simulink model "PVRobusMPC_final"  (R2018a)
settings: Solver=ode2  StartTime=0.0  StopTime=43200  FixedStep=1  RelTol=1e-3  EnableMultiTasking=on
InitFcn:
  | load PV_model_data
StopFcn:
  | save results Lambda_UV01 T_PV_Reference Tm_f01 Pout01 Tamb Time
  | clear all
  | load results
  | figure
  | subplot(3,1,1)
  | plot(Time./3600,T_PV_Reference,Time./3600,Tm_f01)
  | legend('PV Temperature Reference','PV Temperature')
  | title('MPC Tracking')
  | ylim([350 380])
  | subplot(3,1,2)
  | plot(Time./3600,Lambda_UV01)
  | ylim([250 450])
  | legend('\lambda_U_V')
  | subplot(3,1,3)
  | plot(Time./3600,Pout01)
  | legend('PV Power')
  | xlabel('Time [hours]')
  | ylabel('Watt')
values from neighbouring files (symbols this model uses):
  Global_tilt_Irr_2_2_12_13_5 = [0.000279 0.000786 0.00115 0.00401 0.0047 0.0102 0.011 0.0195 0.0266 0.0299 0.0338 0.0682 ... (2802 elements, 1401x2)]    [PV_model_data.mat]
  Total_light_absorption_in_polystyren = [0.0148235487596 0.0159326919994 0.0170383922491 0.0181406655151 0.0192395277052 0.0203349946285 0.0214270819969 0.0225158054254 0.0236011804327 0.0246832224425 0.0257619467839 0.0264640052027 ... (1151 elements, 1151x1)]    [PV_model_data.mat]
  Total_light_absorption_in_PV_cell_acrylic = [0.0222539070262 0.0239185757929 0.0255780524095 0.0272323791236 0.0288816001883 0.030525761736 0.0321649116541 0.0337990994657 0.0354283762117 0.0370527943369 0.0386724075795 0.0397267002838 ... (1151 elements, 1151x1)]    [PV_model_data.mat]
libraries: mpclib x256
(part 1 of 72)
settings Model: Creator=hg212  LastModifiedBy=Mehdi
settings DataIOCC: LimitDataPoints=on  SaveFormat=Array  SignalLoggingSaveFormat=ModelDataLogs
settings OptimizationCC: LifeSpan=inf
settings DebuggingCC: FcnCallInpInsideContextMsg=warning  SFUnexpectedBacktrackingDiag=warning  SFNoUnconditionalDefaultTransitionDiag=warning  SFExecutionAtInitializationDiag=none
settings HardwareCC: ProdBitPerPointer=32  ProdBitPerSizeT=32  ProdBitPerPtrDiffT=32  ProdLargestAtomicFloat=None  ProdIntDivRoundTo=Undefined  ProdEndianess=Unspecified  ProdWordSize=32  ProdHWDeviceType=32-bit Generic
settings ModelReferenceCC: PropagateSignalLabelsOutOfModel=off
settings CodeAppCC: StateflowObjectComments=on
settings GRTTargetCC: TargetLangStandard=C89/C90 (ANSI)  GeneratePreprocessorConditionals=Disable all  CombineOutputUpdateFcns=off  GRTInterface=on
settings ConfigComp: CovMetricSettings=dw  CovHtmlReporting=on  CovSaveCumulativeToWorkspaceVar=on  CovSaveSingleToWorkspaceVar=on  CovExternalEMLEnable=off

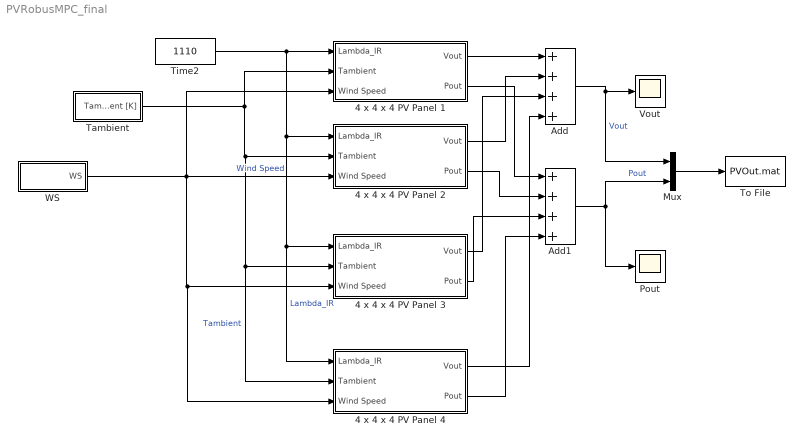
== system PVRobusMPC_final ==
  4 x 4 x 4 PV Panel 1 : Subsystem
  4 x 4 x 4 PV Panel 2 : Subsystem
  4 x 4 x 4 PV Panel 3 : Subsystem
  4 x 4 x 4 PV Panel 4 : Subsystem
  Add : Sum  Inputs=++++
  Add1 : Sum  Inputs=++++
  Mux : Mux  Inputs=2
  Pout : Scope
  Tambient : Subsystem
  Time2 : Constant  Value=1110
  To File : ToFile  Filename=PVOut.mat  SaveFormat=Timeseries
  Vout : Scope
  WS : Subsystem
  wires:
  Time2/1 -> 4 x 4 x 4 PV Panel 4/1(Lambda_IR), 4 x 4 x 4 PV Panel 3/1(Lambda_IR), 4 x 4 x 4 PV Panel 2/1(Lambda_IR), 4 x 4 x 4 PV Panel 1/1(Lambda_IR)  "Lambda_IR"
  Tambient/1(Tambient [K]) -> 4 x 4 x 4 PV Panel 1/2(Tambient), 4 x 4 x 4 PV Panel 4/2(Tambient), 4 x 4 x 4 PV Panel 3/2(Tambient), 4 x 4 x 4 PV Panel 2/2(Tambient)  "Tambient"
  WS/1(WS) -> 4 x 4 x 4 PV Panel 4/3(Wind Speed), 4 x 4 x 4 PV Panel 3/3(Wind Speed), 4 x 4 x 4 PV Panel 2/3(Wind Speed), 4 x 4 x 4 PV Panel 1/3(Wind Speed)  "Wind Speed"
  4 x 4 x 4 PV Panel 1/1(Vout) -> Add/1
  4 x 4 x 4 PV Panel 2/1(Vout) -> Add/2
  4 x 4 x 4 PV Panel 1/2(Pout) -> Add1/1
  4 x 4 x 4 PV Panel 2/2(Pout) -> Add1/2
  Add/1 -> Mux/1, Vout/1  "Vout"
  Add1/1 -> Pout/1, Mux/2  "Pout"
  Mux/1 -> To File/1
  4 x 4 x 4 PV Panel 3/1(Vout) -> Add/3
  4 x 4 x 4 PV Panel 4/1(Vout) -> Add/4
  4 x 4 x 4 PV Panel 3/2(Pout) -> Add1/3
  4 x 4 x 4 PV Panel 4/2(Pout) -> Add1/4

== system PVRobusMPC_final/4 x 4 x 4 PV Panel 1 ==
  Lambda_IR : Inport
  Tambient : Inport  Port=2
  Wind Speed : Inport  Port=3
  4 x 4 PV Panel 1 : Subsystem
  4 x 4 PV Panel 2 : Subsystem
  4 x 4 PV Panel 3 : Subsystem
  4 x 4 PV Panel 4 : Subsystem
  Add : Sum  Inputs=++++
  Add1 : Sum  Inputs=++++
  Vout : Outport
  Pout : Outport  Port=2
  wires:
  4 x 4 PV Panel 2/1(Vout) -> Add/2
  4 x 4 PV Panel 2/2(Pout) -> Add1/2
  4 x 4 PV Panel 4/1(Vout) -> Add/4
  Tambient/1 -> 4 x 4 PV Panel 2/2(Tambient), 4 x 4 PV Panel 4/2(Tambient), 4 x 4 PV Panel 3/2(Tambient), 4 x 4 PV Panel 1/2(Tambient)
  Add1/1 -> Pout/1
  4 x 4 PV Panel 3/1(Vout) -> Add/3
  Lambda_IR/1 -> 4 x 4 PV Panel 4/1(Lambda_IR), 4 x 4 PV Panel 3/1(Lambda_IR), 4 x 4 PV Panel 2/1(Lambda_IR), 4 x 4 PV Panel 1/1(Lambda_IR)
  4 x 4 PV Panel 1/1(Vout) -> Add/1
  4 x 4 PV Panel 4/2(Pout) -> Add1/4
  Wind Speed/1 -> 4 x 4 PV Panel 2/3(Wind Speed), 4 x 4 PV Panel 4/3(Wind Speed), 4 x 4 PV Panel 3/3(Wind Speed), 4 x 4 PV Panel 1/3(Wind Speed)
  4 x 4 PV Panel 3/2(Pout) -> Add1/3
  4 x 4 PV Panel 1/2(Pout) -> Add1/1
  Add/1 -> Vout/1

== system PVRobusMPC_final/4 x 4 x 4 PV Panel 2 ==
  Lambda_IR : Inport
  Tambient : Inport  Port=2
  Wind Speed : Inport  Port=3
  4 x 4 PV Panel 5 : Subsystem
  4 x 4 PV Panel 6 : Subsystem
  4 x 4 PV Panel 7 : Subsystem
  4 x 4 PV Panel 8 : Subsystem
  Add2 : Sum  Inputs=++++
  Add3 : Sum  Inputs=++++
  Vout : Outport
  Pout : Outport  Port=2
  wires:
  Wind Speed/1 -> 4 x 4 PV Panel 8/3(Wind Speed), 4 x 4 PV Panel 7/3(Wind Speed), 4 x 4 PV Panel 6/3(Wind Speed), 4 x 4 PV Panel 5/3(Wind Speed)
  Add3/1 -> Pout/1
  Add2/1 -> Vout/1
  4 x 4 PV Panel 6/1(Vout) -> Add2/2
  Lambda_IR/1 -> 4 x 4 PV Panel 8/1(Lambda_IR), 4 x 4 PV Panel 7/1(Lambda_IR), 4 x 4 PV Panel 6/1(Lambda_IR), 4 x 4 PV Panel 5/1(Lambda_IR)
  Tambient/1 -> 4 x 4 PV Panel 8/2(Tambient), 4 x 4 PV Panel 7/2(Tambient), 4 x 4 PV Panel 6/2(Tambient), 4 x 4 PV Panel 5/2(Tambient)
  4 x 4 PV Panel 8/1(Vout) -> Add2/4
  4 x 4 PV Panel 6/2(Pout) -> Add3/2
  4 x 4 PV Panel 5/1(Vout) -> Add2/1
  4 x 4 PV Panel 7/1(Vout) -> Add2/3
  4 x 4 PV Panel 5/2(Pout) -> Add3/1
  4 x 4 PV Panel 7/2(Pout) -> Add3/3
  4 x 4 PV Panel 8/2(Pout) -> Add3/4

== system PVRobusMPC_final/4 x 4 x 4 PV Panel 3 ==
  Lambda_IR : Inport
  Tambient : Inport  Port=2
  Wind Speed : Inport  Port=3
  4 x 4 PV Panel 5 : Subsystem
  4 x 4 PV Panel 6 : Subsystem
  4 x 4 PV Panel 7 : Subsystem
  4 x 4 PV Panel 8 : Subsystem
  Add2 : Sum  Inputs=++++
  Add3 : Sum  Inputs=++++
  Vout : Outport
  Pout : Outport  Port=2
  wires:
  4 x 4 PV Panel 8/2(Pout) -> Add3/4
  4 x 4 PV Panel 7/2(Pout) -> Add3/3
  4 x 4 PV Panel 5/2(Pout) -> Add3/1
  4 x 4 PV Panel 7/1(Vout) -> Add2/3
  4 x 4 PV Panel 5/1(Vout) -> Add2/1
  4 x 4 PV Panel 6/2(Pout) -> Add3/2
  4 x 4 PV Panel 8/1(Vout) -> Add2/4
  Tambient/1 -> 4 x 4 PV Panel 5/2(Tambient), 4 x 4 PV Panel 6/2(Tambient), 4 x 4 PV Panel 7/2(Tambient), 4 x 4 PV Panel 8/2(Tambient)
  Lambda_IR/1 -> 4 x 4 PV Panel 5/1(Lambda_IR), 4 x 4 PV Panel 6/1(Lambda_IR), 4 x 4 PV Panel 7/1(Lambda_IR), 4 x 4 PV Panel 8/1(Lambda_IR)
  4 x 4 PV Panel 6/1(Vout) -> Add2/2
  Add2/1 -> Vout/1
  Add3/1 -> Pout/1
  Wind Speed/1 -> 4 x 4 PV Panel 5/3(Wind Speed), 4 x 4 PV Panel 6/3(Wind Speed), 4 x 4 PV Panel 7/3(Wind Speed), 4 x 4 PV Panel 8/3(Wind Speed)

== system PVRobusMPC_final/4 x 4 x 4 PV Panel 4 ==
  Lambda_IR : Inport
  Tambient : Inport  Port=2
  Wind Speed : Inport  Port=3
  4 x 4 PV Panel 5 : Subsystem
  4 x 4 PV Panel 6 : Subsystem
  4 x 4 PV Panel 7 : Subsystem
  4 x 4 PV Panel 8 : Subsystem
  Add2 : Sum  Inputs=++++
  Add3 : Sum  Inputs=++++
  Vout : Outport
  Pout : Outport  Port=2
  wires:
  Wind Speed/1 -> 4 x 4 PV Panel 8/3(Wind Speed), 4 x 4 PV Panel 7/3(Wind Speed), 4 x 4 PV Panel 6/3(Wind Speed), 4 x 4 PV Panel 5/3(Wind Speed)
  Add3/1 -> Pout/1
  Add2/1 -> Vout/1
  4 x 4 PV Panel 6/1(Vout) -> Add2/2
  Lambda_IR/1 -> 4 x 4 PV Panel 8/1(Lambda_IR), 4 x 4 PV Panel 7/1(Lambda_IR), 4 x 4 PV Panel 6/1(Lambda_IR), 4 x 4 PV Panel 5/1(Lambda_IR)
  Tambient/1 -> 4 x 4 PV Panel 8/2(Tambient), 4 x 4 PV Panel 7/2(Tambient), 4 x 4 PV Panel 6/2(Tambient), 4 x 4 PV Panel 5/2(Tambient)
  4 x 4 PV Panel 8/1(Vout) -> Add2/4
  4 x 4 PV Panel 6/2(Pout) -> Add3/2
  4 x 4 PV Panel 5/1(Vout) -> Add2/1
  4 x 4 PV Panel 7/1(Vout) -> Add2/3
  4 x 4 PV Panel 5/2(Pout) -> Add3/1
  4 x 4 PV Panel 7/2(Pout) -> Add3/3
  4 x 4 PV Panel 8/2(Pout) -> Add3/4

== system PVRobusMPC_final/Tambient ==
  1-D Lookup Table2 : Lookup_n-D  NumberOfTableDimensions=1  BreakpointsForDimension1=0:600:144*600  Table="[18.16\t18.09\t17.96\t17.97\t18.07\t18.01\t17.98\t17.87\t17.72\t17.76\t17.8\t17.7\t17.54\t17.55\t17.41\t17.38\t17.34\t17.47\t17.23\t17.27\t17.23\t17.29\t17.27\t17.32\t17.27\t17.31\t17.25\t17.48\t17.42\t17.19\t17.16\t17.27\t17.02\t17.11\t17.16\t17.33\t17.27\t17.02\t17\t16.95\t16.96\t16.94\t16.8\t16.73\t16.57\t16.42\t16.64\t16.68\t16.7\t16.94\t17.23\t17.51\t17.41\t17.47\t17.5\t17.69\t17.69\t18.18\t17.97\t17.71\t17.72\t17.83\t18.18\t18.64\t18.99\t18.7\t18.92\t18.9\t19.85\t20.72\t20.99\t20.74\t20.32\t20.88\t21.21\t20.34\t21.6\t20.68\t21.32\t22\t20.4\t21.32\t20.42\t20.54\t22.31\t21.62\t21.9\t20.73\t21.21\t22.06\t22.15\t21.67\t22.11\t21.42\t22.21\t22.47\t23.13\t22.24\t22.02\t21.92\t21.14\t21.67\t21.89\t22.18\t22.28\t21.16\t22.06\t20.81\t20.78\t21.13\t21.15\t20.81\t20.83\t21.02\t20.89\t20.71\t20.73\t20.45\t20.42\t20.09\t20.26\t19.9\t19.45\t19.31\t19.32\t19.1\t18.94\t18.94\t18.8\t18.72\t18.59\t18.5\t18.44\t18.49\t18.46\t18.45\t18.56\t18.32\t18.08\t17.93\t17.79\t17.56\t17.54\t17.23\t17.07]+30+273"  InternalRulePriority=Speed  RndMeth=Simplest  InputSameDT=on
  Clock : Clock
  To Workspace3 : ToWorkspace  VariableName=Tamb  SampleTime=1
  To Workspace7 : ToWorkspace  VariableName=Time  SampleTime=1
  Tambient [K] : Outport
  wires:
  1-D Lookup Table2/1 -> Tambient [K]/1, To Workspace3/1
  Clock/1 -> To Workspace7/1, 1-D Lookup Table2/1

== system PVRobusMPC_final/WS ==
  1-D Lookup Table3 : Lookup_n-D  NumberOfTableDimensions=1  BreakpointsForDimension1=0:600:144*600  Table="[8\t7\t8\t7\t7\t8\t7\t7\t5\t6\t7\t7\t7\t7\t6\t7\t6\t7\t6\t5\t5\t6\t6\t5\t6\t6\t7\t7\t7\t6\t6\t6\t6\t6\t6\t7\t7\t7\t6\t7\t5\t6\t7\t6\t6\t5\t7\t7\t5\t5\t6\t6\t7\t7\t7\t7\t7\t7\t6\t6\t7\t7\t6\t7\t7\t7\t7\t7\t7\t8\t8\t8\t8\t7\t8\t7\t8\t9\t8\t7\t8\t7\t8\t6\t9\t9\t9\t10\t7\t8\t8\t8\t9\t8\t9\t9\t8\t9\t8\t9\t9\t7\t8\t8\t8\t9\t8\t8\t8\t8\t7\t8\t7\t8\t7\t7\t7\t8\t8\t8\t7\t7\t8\t7\t7\t6\t6\t7\t6\t5\t6\t6\t6\t5\t5\t5\t6\t6\t5\t5\t5\t4\t5\t4\t4].*0.277/5"  InternalRulePriority=Speed  RndMeth=Simplest  InputSameDT=on
  Clock1 : Clock
  To Workspace4 : ToWorkspace  VariableName=WS  SampleTime=1
  WS : Outport
  wires:
  Clock1/1 -> 1-D Lookup Table3/1
  1-D Lookup Table3/1 -> WS/1, To Workspace4/1

== system PVRobusMPC_final/4 x 4 x 4 PV Panel 1/4 x 4 PV Panel 1 ==
  Lambda_IR : Inport
  Tambient : Inport  Port=2
  Wind Speed : Inport  Port=3
  4 PV Panel 1 : Subsystem
  4 PV Panel 2 : Subsystem
  4 PV Panel 3 : Subsystem
  4 PV Panel 4 : Subsystem
  Add : Sum  Inputs=++++
  Add2 : Sum  Inputs=++++
  Vout : Outport
  Pout : Outport  Port=2
  wires:
  Wind Speed/1 -> 4 PV Panel 1/3(Wind Speed), 4 PV Panel 2/3(Wind Speed), 4 PV Panel 4/3(Wind Speed), 4 PV Panel 3/3(Wind Speed)
  4 PV Panel 3/2(Pout) -> Add2/3
  4 PV Panel 4/2(Pout) -> Add2/4
  4 PV Panel 3/1(Vout) -> Add/3
  4 PV Panel 2/2(Pout) -> Add2/2
  4 PV Panel 1/1(Vout) -> Add/1
  4 PV Panel 1/2(Pout) -> Add2/1
  Lambda_IR/1 -> 4 PV Panel 4/1(lambda_IR), 4 PV Panel 3/1(lambda_IR), 4 PV Panel 2/1(lambda_IR), 4 PV Panel 1/1(lambda_IR)
  4 PV Panel 4/1(Vout) -> Add/4
  Tambient/1 -> 4 PV Panel 1/2(Tambient1), 4 PV Panel 4/2(Tambient), 4 PV Panel 3/2(Tambient), 4 PV Panel 2/2(Tambient)
  4 PV Panel 2/1(Vout) -> Add/2
  Add2/1 -> Pout/1
  Add/1 -> Vout/1

== system PVRobusMPC_final/4 x 4 x 4 PV Panel 1/4 x 4 PV Panel 2 ==
  Lambda_IR : Inport
  Tambient : Inport  Port=2
  Wind Speed : Inport  Port=3
  4 PV Panel 1 : Subsystem
  4 PV Panel 2 : Subsystem
  4 PV Panel 3 : Subsystem
  4 PV Panel 4 : Subsystem
  Add : Sum  Inputs=++++
  Add2 : Sum  Inputs=++++
  Vout : Outport
  Pout : Outport  Port=2
  wires:
  Add/1 -> Vout/1
  Add2/1 -> Pout/1
  4 PV Panel 2/1(Vout) -> Add/2
  Tambient/1 -> 4 PV Panel 2/2(Tambient), 4 PV Panel 3/2(Tambient), 4 PV Panel 4/2(Tambient), 4 PV Panel 1/2(Tambient1)
  4 PV Panel 4/1(Vout) -> Add/4
  Lambda_IR/1 -> 4 PV Panel 1/1(lambda_IR), 4 PV Panel 2/1(lambda_IR), 4 PV Panel 3/1(lambda_IR), 4 PV Panel 4/1(lambda_IR)
  4 PV Panel 1/2(Pout) -> Add2/1
  4 PV Panel 1/1(Vout) -> Add/1
  4 PV Panel 2/2(Pout) -> Add2/2
  4 PV Panel 3/1(Vout) -> Add/3
  4 PV Panel 4/2(Pout) -> Add2/4
  4 PV Panel 3/2(Pout) -> Add2/3
  Wind Speed/1 -> 4 PV Panel 3/3(Wind Speed), 4 PV Panel 4/3(Wind Speed), 4 PV Panel 2/3(Wind Speed), 4 PV Panel 1/3(Wind Speed)

== system PVRobusMPC_final/4 x 4 x 4 PV Panel 1/4 x 4 PV Panel 3 ==
  Lambda_IR : Inport
  Tambient : Inport  Port=2
  Wind Speed : Inport  Port=3
  4 PV Panel 1 : Subsystem
  4 PV Panel 2 : Subsystem
  4 PV Panel 3 : Subsystem
  4 PV Panel 4 : Subsystem
  Add : Sum  Inputs=++++
  Add2 : Sum  Inputs=++++
  Vout : Outport
  Pout : Outport  Port=2
  wires:
  Add/1 -> Vout/1
  Add2/1 -> Pout/1
  4 PV Panel 2/1(Vout) -> Add/2
  Tambient/1 -> 4 PV Panel 2/2(Tambient), 4 PV Panel 3/2(Tambient), 4 PV Panel 4/2(Tambient), 4 PV Panel 1/2(Tambient1)
  4 PV Panel 4/1(Vout) -> Add/4
  Lambda_IR/1 -> 4 PV Panel 1/1(lambda_IR), 4 PV Panel 2/1(lambda_IR), 4 PV Panel 3/1(lambda_IR), 4 PV Panel 4/1(lambda_IR)
  4 PV Panel 1/2(Pout) -> Add2/1
  4 PV Panel 1/1(Vout) -> Add/1
  4 PV Panel 2/2(Pout) -> Add2/2
  4 PV Panel 3/1(Vout) -> Add/3
  4 PV Panel 4/2(Pout) -> Add2/4
  4 PV Panel 3/2(Pout) -> Add2/3
  Wind Speed/1 -> 4 PV Panel 3/3(Wind Speed), 4 PV Panel 4/3(Wind Speed), 4 PV Panel 2/3(Wind Speed), 4 PV Panel 1/3(Wind Speed)

== system PVRobusMPC_final/4 x 4 x 4 PV Panel 1/4 x 4 PV Panel 4 ==
  Lambda_IR : Inport
  Tambient : Inport  Port=2
  Wind Speed : Inport  Port=3
  4 PV Panel 1 : Subsystem
  4 PV Panel 2 : Subsystem
  4 PV Panel 3 : Subsystem
  4 PV Panel 4 : Subsystem
  Add : Sum  Inputs=++++
  Add2 : Sum  Inputs=++++
  Vout : Outport
  Pout : Outport  Port=2
  wires:
  Add/1 -> Vout/1
  Add2/1 -> Pout/1
  4 PV Panel 2/1(Vout) -> Add/2
  Tambient/1 -> 4 PV Panel 2/2(Tambient), 4 PV Panel 3/2(Tambient), 4 PV Panel 4/2(Tambient), 4 PV Panel 1/2(Tambient1)
  4 PV Panel 4/1(Vout) -> Add/4
  Lambda_IR/1 -> 4 PV Panel 1/1(lambda_IR), 4 PV Panel 2/1(lambda_IR), 4 PV Panel 3/1(lambda_IR), 4 PV Panel 4/1(lambda_IR)
  4 PV Panel 1/2(Pout) -> Add2/1
  4 PV Panel 1/1(Vout) -> Add/1
  4 PV Panel 2/2(Pout) -> Add2/2
  4 PV Panel 3/1(Vout) -> Add/3
  4 PV Panel 4/2(Pout) -> Add2/4
  4 PV Panel 3/2(Pout) -> Add2/3
  Wind Speed/1 -> 4 PV Panel 3/3(Wind Speed), 4 PV Panel 4/3(Wind Speed), 4 PV Panel 2/3(Wind Speed), 4 PV Panel 1/3(Wind Speed)

== system PVRobusMPC_final/4 x 4 x 4 PV Panel 2/4 x 4 PV Panel 5 ==
  Lambda_IR : Inport
  Tambient : Inport  Port=2
  Wind Speed : Inport  Port=3
  4 PV Panel 1 : Subsystem
  4 PV Panel 2 : Subsystem
  4 PV Panel 3 : Subsystem
  4 PV Panel 4 : Subsystem
  Add : Sum  Inputs=++++
  Add2 : Sum  Inputs=++++
  Vout : Outport
  Pout : Outport  Port=2
  wires:
  Wind Speed/1 -> 4 PV Panel 1/3(Wind Speed), 4 PV Panel 2/3(Wind Speed), 4 PV Panel 4/3(Wind Speed), 4 PV Panel 3/3(Wind Speed)
  4 PV Panel 3/2(Pout) -> Add2/3
  4 PV Panel 4/2(Pout) -> Add2/4
  4 PV Panel 3/1(Vout) -> Add/3
  4 PV Panel 2/2(Pout) -> Add2/2
  4 PV Panel 1/1(Vout) -> Add/1
  4 PV Panel 1/2(Pout) -> Add2/1
  Lambda_IR/1 -> 4 PV Panel 4/1(lambda_IR), 4 PV Panel 3/1(lambda_IR), 4 PV Panel 2/1(lambda_IR), 4 PV Panel 1/1(lambda_IR)
  4 PV Panel 4/1(Vout) -> Add/4
  Tambient/1 -> 4 PV Panel 1/2(Tambient1), 4 PV Panel 4/2(Tambient), 4 PV Panel 3/2(Tambient), 4 PV Panel 2/2(Tambient)
  4 PV Panel 2/1(Vout) -> Add/2
  Add2/1 -> Pout/1
  Add/1 -> Vout/1

== system PVRobusMPC_final/4 x 4 x 4 PV Panel 2/4 x 4 PV Panel 6 ==
  Lambda_IR : Inport
  Tambient : Inport  Port=2
  Wind Speed : Inport  Port=3
  4 PV Panel 1 : Subsystem
  4 PV Panel 2 : Subsystem
  4 PV Panel 3 : Subsystem
  4 PV Panel 4 : Subsystem
  Add : Sum  Inputs=++++
  Add2 : Sum  Inputs=++++
  Vout : Outport
  Pout : Outport  Port=2
  wires:
  Wind Speed/1 -> 4 PV Panel 1/3(Wind Speed), 4 PV Panel 2/3(Wind Speed), 4 PV Panel 4/3(Wind Speed), 4 PV Panel 3/3(Wind Speed)
  4 PV Panel 3/2(Pout) -> Add2/3
  4 PV Panel 4/2(Pout) -> Add2/4
  4 PV Panel 3/1(Vout) -> Add/3
  4 PV Panel 2/2(Pout) -> Add2/2
  4 PV Panel 1/1(Vout) -> Add/1
  4 PV Panel 1/2(Pout) -> Add2/1
  Lambda_IR/1 -> 4 PV Panel 4/1(lambda_IR), 4 PV Panel 3/1(lambda_IR), 4 PV Panel 2/1(lambda_IR), 4 PV Panel 1/1(lambda_IR)
  4 PV Panel 4/1(Vout) -> Add/4
  Tambient/1 -> 4 PV Panel 1/2(Tambient1), 4 PV Panel 4/2(Tambient), 4 PV Panel 3/2(Tambient), 4 PV Panel 2/2(Tambient)
  4 PV Panel 2/1(Vout) -> Add/2
  Add2/1 -> Pout/1
  Add/1 -> Vout/1

== system PVRobusMPC_final/4 x 4 x 4 PV Panel 2/4 x 4 PV Panel 7 ==
  Lambda_IR : Inport
  Tambient : Inport  Port=2
  Wind Speed : Inport  Port=3
  4 PV Panel 1 : Subsystem
  4 PV Panel 2 : Subsystem
  4 PV Panel 3 : Subsystem
  4 PV Panel 4 : Subsystem
  Add : Sum  Inputs=++++
  Add2 : Sum  Inputs=++++
  Vout : Outport
  Pout : Outport  Port=2
  wires:
  Wind Speed/1 -> 4 PV Panel 1/3(Wind Speed), 4 PV Panel 2/3(Wind Speed), 4 PV Panel 4/3(Wind Speed), 4 PV Panel 3/3(Wind Speed)
  4 PV Panel 3/2(Pout) -> Add2/3
  4 PV Panel 4/2(Pout) -> Add2/4
  4 PV Panel 3/1(Vout) -> Add/3
  4 PV Panel 2/2(Pout) -> Add2/2
  4 PV Panel 1/1(Vout) -> Add/1
  4 PV Panel 1/2(Pout) -> Add2/1
  Lambda_IR/1 -> 4 PV Panel 4/1(lambda_IR), 4 PV Panel 3/1(lambda_IR), 4 PV Panel 2/1(lambda_IR), 4 PV Panel 1/1(lambda_IR)
  4 PV Panel 4/1(Vout) -> Add/4
  Tambient/1 -> 4 PV Panel 1/2(Tambient1), 4 PV Panel 4/2(Tambient), 4 PV Panel 3/2(Tambient), 4 PV Panel 2/2(Tambient)
  4 PV Panel 2/1(Vout) -> Add/2
  Add2/1 -> Pout/1
  Add/1 -> Vout/1

== system PVRobusMPC_final/4 x 4 x 4 PV Panel 2/4 x 4 PV Panel 8 ==
  Lambda_IR : Inport
  Tambient : Inport  Port=2
  Wind Speed : Inport  Port=3
  4 PV Panel 1 : Subsystem
  4 PV Panel 2 : Subsystem
  4 PV Panel 3 : Subsystem
  4 PV Panel 4 : Subsystem
  Add : Sum  Inputs=++++
  Add2 : Sum  Inputs=++++
  Vout : Outport
  Pout : Outport  Port=2
  wires:
  Add/1 -> Vout/1
  Add2/1 -> Pout/1
  4 PV Panel 2/1(Vout) -> Add/2
  Tambient/1 -> 4 PV Panel 2/2(Tambient), 4 PV Panel 3/2(Tambient), 4 PV Panel 4/2(Tambient), 4 PV Panel 1/2(Tambient1)
  4 PV Panel 4/1(Vout) -> Add/4
  Lambda_IR/1 -> 4 PV Panel 1/1(lambda_IR), 4 PV Panel 2/1(lambda_IR), 4 PV Panel 3/1(lambda_IR), 4 PV Panel 4/1(lambda_IR)
  4 PV Panel 1/2(Pout) -> Add2/1
  4 PV Panel 1/1(Vout) -> Add/1
  4 PV Panel 2/2(Pout) -> Add2/2
  4 PV Panel 3/1(Vout) -> Add/3
  4 PV Panel 4/2(Pout) -> Add2/4
  4 PV Panel 3/2(Pout) -> Add2/3
  Wind Speed/1 -> 4 PV Panel 3/3(Wind Speed), 4 PV Panel 4/3(Wind Speed), 4 PV Panel 2/3(Wind Speed), 4 PV Panel 1/3(Wind Speed)

== system PVRobusMPC_final/4 x 4 x 4 PV Panel 3/4 x 4 PV Panel 5 ==
  Lambda_IR : Inport
  Tambient : Inport  Port=2
  Wind Speed : Inport  Port=3
  4 PV Panel 1 : Subsystem
  4 PV Panel 2 : Subsystem
  4 PV Panel 3 : Subsystem
  4 PV Panel 4 : Subsystem
  Add : Sum  Inputs=++++
  Add2 : Sum  Inputs=++++
  Vout : Outport
  Pout : Outport  Port=2
  wires:
  Add/1 -> Vout/1
  Add2/1 -> Pout/1
  4 PV Panel 2/1(Vout) -> Add/2
  Tambient/1 -> 4 PV Panel 2/2(Tambient), 4 PV Panel 3/2(Tambient), 4 PV Panel 4/2(Tambient), 4 PV Panel 1/2(Tambient1)
  4 PV Panel 4/1(Vout) -> Add/4
  Lambda_IR/1 -> 4 PV Panel 1/1(lambda_IR), 4 PV Panel 2/1(lambda_IR), 4 PV Panel 3/1(lambda_IR), 4 PV Panel 4/1(lambda_IR)
  4 PV Panel 1/2(Pout) -> Add2/1
  4 PV Panel 1/1(Vout) -> Add/1
  4 PV Panel 2/2(Pout) -> Add2/2
  4 PV Panel 3/1(Vout) -> Add/3
  4 PV Panel 4/2(Pout) -> Add2/4
  4 PV Panel 3/2(Pout) -> Add2/3
  Wind Speed/1 -> 4 PV Panel 3/3(Wind Speed), 4 PV Panel 4/3(Wind Speed), 4 PV Panel 2/3(Wind Speed), 4 PV Panel 1/3(Wind Speed)

== system PVRobusMPC_final/4 x 4 x 4 PV Panel 3/4 x 4 PV Panel 6 ==
  Lambda_IR : Inport
  Tambient : Inport  Port=2
  Wind Speed : Inport  Port=3
  4 PV Panel 1 : Subsystem
  4 PV Panel 2 : Subsystem
  4 PV Panel 3 : Subsystem
  4 PV Panel 4 : Subsystem
  Add : Sum  Inputs=++++
  Add2 : Sum  Inputs=++++
  Vout : Outport
  Pout : Outport  Port=2
  wires:
  Add/1 -> Vout/1
  Add2/1 -> Pout/1
  4 PV Panel 2/1(Vout) -> Add/2
  Tambient/1 -> 4 PV Panel 2/2(Tambient), 4 PV Panel 3/2(Tambient), 4 PV Panel 4/2(Tambient), 4 PV Panel 1/2(Tambient1)
  4 PV Panel 4/1(Vout) -> Add/4
  Lambda_IR/1 -> 4 PV Panel 1/1(lambda_IR), 4 PV Panel 2/1(lambda_IR), 4 PV Panel 3/1(lambda_IR), 4 PV Panel 4/1(lambda_IR)
  4 PV Panel 1/2(Pout) -> Add2/1
  4 PV Panel 1/1(Vout) -> Add/1
  4 PV Panel 2/2(Pout) -> Add2/2
  4 PV Panel 3/1(Vout) -> Add/3
  4 PV Panel 4/2(Pout) -> Add2/4
  4 PV Panel 3/2(Pout) -> Add2/3
  Wind Speed/1 -> 4 PV Panel 3/3(Wind Speed), 4 PV Panel 4/3(Wind Speed), 4 PV Panel 2/3(Wind Speed), 4 PV Panel 1/3(Wind Speed)

== system PVRobusMPC_final/4 x 4 x 4 PV Panel 3/4 x 4 PV Panel 7 ==
  Lambda_IR : Inport
  Tambient : Inport  Port=2
  Wind Speed : Inport  Port=3
  4 PV Panel 1 : Subsystem
  4 PV Panel 2 : Subsystem
  4 PV Panel 3 : Subsystem
  4 PV Panel 4 : Subsystem
  Add : Sum  Inputs=++++
  Add2 : Sum  Inputs=++++
  Vout : Outport
  Pout : Outport  Port=2
  wires:
  Add/1 -> Vout/1
  Add2/1 -> Pout/1
  4 PV Panel 2/1(Vout) -> Add/2
  Tambient/1 -> 4 PV Panel 2/2(Tambient), 4 PV Panel 3/2(Tambient), 4 PV Panel 4/2(Tambient), 4 PV Panel 1/2(Tambient1)
  4 PV Panel 4/1(Vout) -> Add/4
  Lambda_IR/1 -> 4 PV Panel 1/1(lambda_IR), 4 PV Panel 2/1(lambda_IR), 4 PV Panel 3/1(lambda_IR), 4 PV Panel 4/1(lambda_IR)
  4 PV Panel 1/2(Pout) -> Add2/1
  4 PV Panel 1/1(Vout) -> Add/1
  4 PV Panel 2/2(Pout) -> Add2/2
  4 PV Panel 3/1(Vout) -> Add/3
  4 PV Panel 4/2(Pout) -> Add2/4
  4 PV Panel 3/2(Pout) -> Add2/3
  Wind Speed/1 -> 4 PV Panel 3/3(Wind Speed), 4 PV Panel 4/3(Wind Speed), 4 PV Panel 2/3(Wind Speed), 4 PV Panel 1/3(Wind Speed)

== system PVRobusMPC_final/4 x 4 x 4 PV Panel 3/4 x 4 PV Panel 8 ==
  Lambda_IR : Inport
  Tambient : Inport  Port=2
  Wind Speed : Inport  Port=3
  4 PV Panel 1 : Subsystem
  4 PV Panel 2 : Subsystem
  4 PV Panel 3 : Subsystem
  4 PV Panel 4 : Subsystem
  Add : Sum  Inputs=++++
  Add2 : Sum  Inputs=++++
  Vout : Outport
  Pout : Outport  Port=2
  wires:
  Wind Speed/1 -> 4 PV Panel 1/3(Wind Speed), 4 PV Panel 2/3(Wind Speed), 4 PV Panel 4/3(Wind Speed), 4 PV Panel 3/3(Wind Speed)
  4 PV Panel 3/2(Pout) -> Add2/3
  4 PV Panel 4/2(Pout) -> Add2/4
  4 PV Panel 3/1(Vout) -> Add/3
  4 PV Panel 2/2(Pout) -> Add2/2
  4 PV Panel 1/1(Vout) -> Add/1
  4 PV Panel 1/2(Pout) -> Add2/1
  Lambda_IR/1 -> 4 PV Panel 4/1(lambda_IR), 4 PV Panel 3/1(lambda_IR), 4 PV Panel 2/1(lambda_IR), 4 PV Panel 1/1(lambda_IR)
  4 PV Panel 4/1(Vout) -> Add/4
  Tambient/1 -> 4 PV Panel 1/2(Tambient1), 4 PV Panel 4/2(Tambient), 4 PV Panel 3/2(Tambient), 4 PV Panel 2/2(Tambient)
  4 PV Panel 2/1(Vout) -> Add/2
  Add2/1 -> Pout/1
  Add/1 -> Vout/1

== system PVRobusMPC_final/4 x 4 x 4 PV Panel 4/4 x 4 PV Panel 5 ==
  Lambda_IR : Inport
  Tambient : Inport  Port=2
  Wind Speed : Inport  Port=3
  4 PV Panel 1 : Subsystem
  4 PV Panel 2 : Subsystem
  4 PV Panel 3 : Subsystem
  4 PV Panel 4 : Subsystem
  Add : Sum  Inputs=++++
  Add2 : Sum  Inputs=++++
  Vout : Outport
  Pout : Outport  Port=2
  wires:
  Wind Speed/1 -> 4 PV Panel 1/3(Wind Speed), 4 PV Panel 2/3(Wind Speed), 4 PV Panel 4/3(Wind Speed), 4 PV Panel 3/3(Wind Speed)
  4 PV Panel 3/2(Pout) -> Add2/3
  4 PV Panel 4/2(Pout) -> Add2/4
  4 PV Panel 3/1(Vout) -> Add/3
  4 PV Panel 2/2(Pout) -> Add2/2
  4 PV Panel 1/1(Vout) -> Add/1
  4 PV Panel 1/2(Pout) -> Add2/1
  Lambda_IR/1 -> 4 PV Panel 4/1(lambda_IR), 4 PV Panel 3/1(lambda_IR), 4 PV Panel 2/1(lambda_IR), 4 PV Panel 1/1(lambda_IR)
  4 PV Panel 4/1(Vout) -> Add/4
  Tambient/1 -> 4 PV Panel 1/2(Tambient1), 4 PV Panel 4/2(Tambient), 4 PV Panel 3/2(Tambient), 4 PV Panel 2/2(Tambient)
  4 PV Panel 2/1(Vout) -> Add/2
  Add2/1 -> Pout/1
  Add/1 -> Vout/1

== system PVRobusMPC_final/4 x 4 x 4 PV Panel 4/4 x 4 PV Panel 6 ==
  Lambda_IR : Inport
  Tambient : Inport  Port=2
  Wind Speed : Inport  Port=3
  4 PV Panel 1 : Subsystem
  4 PV Panel 2 : Subsystem
  4 PV Panel 3 : Subsystem
  4 PV Panel 4 : Subsystem
  Add : Sum  Inputs=++++
  Add2 : Sum  Inputs=++++
  Vout : Outport
  Pout : Outport  Port=2
  wires:
  Wind Speed/1 -> 4 PV Panel 1/3(Wind Speed), 4 PV Panel 2/3(Wind Speed), 4 PV Panel 4/3(Wind Speed), 4 PV Panel 3/3(Wind Speed)
  4 PV Panel 3/2(Pout) -> Add2/3
  4 PV Panel 4/2(Pout) -> Add2/4
  4 PV Panel 3/1(Vout) -> Add/3
  4 PV Panel 2/2(Pout) -> Add2/2
  4 PV Panel 1/1(Vout) -> Add/1
  4 PV Panel 1/2(Pout) -> Add2/1
  Lambda_IR/1 -> 4 PV Panel 4/1(lambda_IR), 4 PV Panel 3/1(lambda_IR), 4 PV Panel 2/1(lambda_IR), 4 PV Panel 1/1(lambda_IR)
  4 PV Panel 4/1(Vout) -> Add/4
  Tambient/1 -> 4 PV Panel 1/2(Tambient1), 4 PV Panel 4/2(Tambient), 4 PV Panel 3/2(Tambient), 4 PV Panel 2/2(Tambient)
  4 PV Panel 2/1(Vout) -> Add/2
  Add2/1 -> Pout/1
  Add/1 -> Vout/1

== system PVRobusMPC_final/4 x 4 x 4 PV Panel 4/4 x 4 PV Panel 7 ==
  Lambda_IR : Inport
  Tambient : Inport  Port=2
  Wind Speed : Inport  Port=3
  4 PV Panel 1 : Subsystem
  4 PV Panel 2 : Subsystem
  4 PV Panel 3 : Subsystem
  4 PV Panel 4 : Subsystem
  Add : Sum  Inputs=++++
  Add2 : Sum  Inputs=++++
  Vout : Outport
  Pout : Outport  Port=2
  wires:
  Wind Speed/1 -> 4 PV Panel 1/3(Wind Speed), 4 PV Panel 2/3(Wind Speed), 4 PV Panel 4/3(Wind Speed), 4 PV Panel 3/3(Wind Speed)
  4 PV Panel 3/2(Pout) -> Add2/3
  4 PV Panel 4/2(Pout) -> Add2/4
  4 PV Panel 3/1(Vout) -> Add/3
  4 PV Panel 2/2(Pout) -> Add2/2
  4 PV Panel 1/1(Vout) -> Add/1
  4 PV Panel 1/2(Pout) -> Add2/1
  Lambda_IR/1 -> 4 PV Panel 4/1(lambda_IR), 4 PV Panel 3/1(lambda_IR), 4 PV Panel 2/1(lambda_IR), 4 PV Panel 1/1(lambda_IR)
  4 PV Panel 4/1(Vout) -> Add/4
  Tambient/1 -> 4 PV Panel 1/2(Tambient1), 4 PV Panel 4/2(Tambient), 4 PV Panel 3/2(Tambient), 4 PV Panel 2/2(Tambient)
  4 PV Panel 2/1(Vout) -> Add/2
  Add2/1 -> Pout/1
  Add/1 -> Vout/1

== system PVRobusMPC_final/4 x 4 x 4 PV Panel 4/4 x 4 PV Panel 8 ==
  Lambda_IR : Inport
  Tambient : Inport  Port=2
  Wind Speed : Inport  Port=3
  4 PV Panel 1 : Subsystem
  4 PV Panel 2 : Subsystem
  4 PV Panel 3 : Subsystem
  4 PV Panel 4 : Subsystem
  Add : Sum  Inputs=++++
  Add2 : Sum  Inputs=++++
  Vout : Outport
  Pout : Outport  Port=2
  wires:
  Add/1 -> Vout/1
  Add2/1 -> Pout/1
  4 PV Panel 2/1(Vout) -> Add/2
  Tambient/1 -> 4 PV Panel 2/2(Tambient), 4 PV Panel 3/2(Tambient), 4 PV Panel 4/2(Tambient), 4 PV Panel 1/2(Tambient1)
  4 PV Panel 4/1(Vout) -> Add/4
  Lambda_IR/1 -> 4 PV Panel 1/1(lambda_IR), 4 PV Panel 2/1(lambda_IR), 4 PV Panel 3/1(lambda_IR), 4 PV Panel 4/1(lambda_IR)
  4 PV Panel 1/2(Pout) -> Add2/1
  4 PV Panel 1/1(Vout) -> Add/1
  4 PV Panel 2/2(Pout) -> Add2/2
  4 PV Panel 3/1(Vout) -> Add/3
  4 PV Panel 4/2(Pout) -> Add2/4
  4 PV Panel 3/2(Pout) -> Add2/3
  Wind Speed/1 -> 4 PV Panel 3/3(Wind Speed), 4 PV Panel 4/3(Wind Speed), 4 PV Panel 2/3(Wind Speed), 4 PV Panel 1/3(Wind Speed)

== system PVRobusMPC_final/4 x 4 x 4 PV Panel 1/4 x 4 PV Panel 1/4 PV Panel 1 ==
  lambda_IR : Inport
  Tambient1 : Inport  Port=2
  Wind Speed : Inport  Port=3
  Add : Sum  Inputs=++++
  Add2 : Sum  Inputs=++++
  PV Panel 1 : Subsystem
  PV Panel 2 : Subsystem
  PV Panel 3 : Subsystem
  PV Panel 4 : Subsystem
  Vout : Outport
  Pout : Outport  Port=2
  wires:
  PV Panel 3/2(Pout) -> Add2/3
  lambda_IR/1 -> PV Panel 1/1(Lambda_IR), PV Panel 2/1(Lambda_IR), PV Panel 4/1(Lambda_IR), PV Panel 3/1(Lambda_IR)
  Add/1 -> Vout/1
  PV Panel 1/2(Pout) -> Add2/1
  Tambient1/1 -> PV Panel 1/2(Tambient), PV Panel 2/2(Tambient), PV Panel 3/2(Tambient), PV Panel 4/2(Tambient)
  PV Panel 1/1(Vout) -> Add/1
  PV Panel 4/1(Vout) -> Add/4
  Wind Speed/1 -> PV Panel 1/3(Wind Speed), PV Panel 2/3(Wind Speed), PV Panel 4/3(Wind Speed), PV Panel 3/3(Wind Speed)
  PV Panel 3/1(Vout) -> Add/3
  PV Panel 2/2(Pout) -> Add2/2
  PV Panel 4/2(Pout) -> Add2/4
  PV Panel 2/1(Vout) -> Add/2
  Add2/1 -> Pout/1

== system PVRobusMPC_final/4 x 4 x 4 PV Panel 1/4 x 4 PV Panel 1/4 PV Panel 2 ==
  lambda_IR : Inport
  Tambient : Inport  Port=2
  Wind Speed : Inport  Port=3
  Add1 : Sum  Inputs=++++
  Add3 : Sum  Inputs=++++
  PV Panel 5 : Subsystem
  PV Panel 6 : Subsystem
  PV Panel 7 : Subsystem
  PV Panel 8 : Subsystem
  Vout : Outport
  Pout : Outport  Port=2
  wires:
  PV Panel 5/1(Vout) -> Add1/1
  PV Panel 6/2(Pout) -> Add3/2
  PV Panel 7/1(Vout) -> Add1/3
  Wind Speed/1 -> PV Panel 5/3(Wind Speed), PV Panel 6/3(Wind Speed), PV Panel 8/3(Wind Speed), PV Panel 7/3(Wind Speed)
  Tambient/1 -> PV Panel 5/2(Tambient), PV Panel 6/2(Tambient), PV Panel 8/2(Tambient), PV Panel 7/2(Tambient)
  Add3/1 -> Pout/1
  PV Panel 7/2(Pout) -> Add3/3
  lambda_IR/1 -> PV Panel 6/1(Lambda_IR), PV Panel 8/1(Lambda_IR), PV Panel 7/1(Lambda_IR), PV Panel 5/1(Lambda_IR)
  PV Panel 6/1(Vout) -> Add1/2
  PV Panel 8/1(Vout) -> Add1/4
  Add1/1 -> Vout/1
  PV Panel 8/2(Pout) -> Add3/4
  PV Panel 5/2(Pout) -> Add3/1

== system PVRobusMPC_final/4 x 4 x 4 PV Panel 1/4 x 4 PV Panel 1/4 PV Panel 3 ==
  lambda_IR : Inport
  Tambient : Inport  Port=2
  Wind Speed : Inport  Port=3
  Add1 : Sum  Inputs=++++
  Add3 : Sum  Inputs=++++
  PV Panel 5 : Subsystem
  PV Panel 6 : Subsystem
  PV Panel 7 : Subsystem
  PV Panel 8 : Subsystem
  Vout : Outport
  Pout : Outport  Port=2
  wires:
  PV Panel 5/2(Pout) -> Add3/1
  PV Panel 8/2(Pout) -> Add3/4
  Add1/1 -> Vout/1
  PV Panel 8/1(Vout) -> Add1/4
  PV Panel 6/1(Vout) -> Add1/2
  lambda_IR/1 -> PV Panel 5/1(Lambda_IR), PV Panel 7/1(Lambda_IR), PV Panel 8/1(Lambda_IR), PV Panel 6/1(Lambda_IR)
  PV Panel 7/2(Pout) -> Add3/3
  Add3/1 -> Pout/1
  Tambient/1 -> PV Panel 7/2(Tambient), PV Panel 8/2(Tambient), PV Panel 6/2(Tambient), PV Panel 5/2(Tambient)
  Wind Speed/1 -> PV Panel 7/3(Wind Speed), PV Panel 8/3(Wind Speed), PV Panel 6/3(Wind Speed), PV Panel 5/3(Wind Speed)
  PV Panel 7/1(Vout) -> Add1/3
  PV Panel 6/2(Pout) -> Add3/2
  PV Panel 5/1(Vout) -> Add1/1

== system PVRobusMPC_final/4 x 4 x 4 PV Panel 1/4 x 4 PV Panel 1/4 PV Panel 4 ==
  lambda_IR : Inport
  Tambient : Inport  Port=2
  Wind Speed : Inport  Port=3
  Add1 : Sum  Inputs=++++
  Add3 : Sum  Inputs=++++
  PV Panel 5 : Subsystem
  PV Panel 6 : Subsystem
  PV Panel 7 : Subsystem
  PV Panel 8 : Subsystem
  Vout : Outport
  Pout : Outport  Port=2
  wires:
  PV Panel 5/1(Vout) -> Add1/1
  PV Panel 6/2(Pout) -> Add3/2
  PV Panel 7/1(Vout) -> Add1/3
  Wind Speed/1 -> PV Panel 5/3(Wind Speed), PV Panel 6/3(Wind Speed), PV Panel 8/3(Wind Speed), PV Panel 7/3(Wind Speed)
  Tambient/1 -> PV Panel 5/2(Tambient), PV Panel 6/2(Tambient), PV Panel 8/2(Tambient), PV Panel 7/2(Tambient)
  Add3/1 -> Pout/1
  PV Panel 7/2(Pout) -> Add3/3
  lambda_IR/1 -> PV Panel 6/1(Lambda_IR), PV Panel 8/1(Lambda_IR), PV Panel 7/1(Lambda_IR), PV Panel 5/1(Lambda_IR)
  PV Panel 6/1(Vout) -> Add1/2
  PV Panel 8/1(Vout) -> Add1/4
  Add1/1 -> Vout/1
  PV Panel 8/2(Pout) -> Add3/4
  PV Panel 5/2(Pout) -> Add3/1

== system PVRobusMPC_final/4 x 4 x 4 PV Panel 1/4 x 4 PV Panel 2/4 PV Panel 1 ==
  lambda_IR : Inport
  Tambient1 : Inport  Port=2
  Wind Speed : Inport  Port=3
  Add : Sum  Inputs=++++
  Add2 : Sum  Inputs=++++
  PV Panel 1 : Subsystem
  PV Panel 2 : Subsystem
  PV Panel 3 : Subsystem
  PV Panel 4 : Subsystem
  Vout : Outport
  Pout : Outport  Port=2
  wires:
  Add2/1 -> Pout/1
  PV Panel 2/1(Vout) -> Add/2
  PV Panel 4/2(Pout) -> Add2/4
  PV Panel 2/2(Pout) -> Add2/2
  PV Panel 3/1(Vout) -> Add/3
  Wind Speed/1 -> PV Panel 3/3(Wind Speed), PV Panel 4/3(Wind Speed), PV Panel 2/3(Wind Speed), PV Panel 1/3(Wind Speed)
  PV Panel 4/1(Vout) -> Add/4
  PV Panel 1/1(Vout) -> Add/1
  Tambient1/1 -> PV Panel 4/2(Tambient), PV Panel 3/2(Tambient), PV Panel 2/2(Tambient), PV Panel 1/2(Tambient)
  PV Panel 1/2(Pout) -> Add2/1
  Add/1 -> Vout/1
  lambda_IR/1 -> PV Panel 3/1(Lambda_IR), PV Panel 4/1(Lambda_IR), PV Panel 2/1(Lambda_IR), PV Panel 1/1(Lambda_IR)
  PV Panel 3/2(Pout) -> Add2/3

== system PVRobusMPC_final/4 x 4 x 4 PV Panel 1/4 x 4 PV Panel 2/4 PV Panel 2 ==
  lambda_IR : Inport
  Tambient : Inport  Port=2
  Wind Speed : Inport  Port=3
  Add1 : Sum  Inputs=++++
  Add3 : Sum  Inputs=++++
  PV Panel 5 : Subsystem
  PV Panel 6 : Subsystem
  PV Panel 7 : Subsystem
  PV Panel 8 : Subsystem
  Vout : Outport
  Pout : Outport  Port=2
  wires:
  PV Panel 5/2(Pout) -> Add3/1
  PV Panel 8/2(Pout) -> Add3/4
  Add1/1 -> Vout/1
  PV Panel 8/1(Vout) -> Add1/4
  PV Panel 6/1(Vout) -> Add1/2
  lambda_IR/1 -> PV Panel 5/1(Lambda_IR), PV Panel 7/1(Lambda_IR), PV Panel 8/1(Lambda_IR), PV Panel 6/1(Lambda_IR)
  PV Panel 7/2(Pout) -> Add3/3
  Add3/1 -> Pout/1
  Tambient/1 -> PV Panel 7/2(Tambient), PV Panel 8/2(Tambient), PV Panel 6/2(Tambient), PV Panel 5/2(Tambient)
  Wind Speed/1 -> PV Panel 7/3(Wind Speed), PV Panel 8/3(Wind Speed), PV Panel 6/3(Wind Speed), PV Panel 5/3(Wind Speed)
  PV Panel 7/1(Vout) -> Add1/3
  PV Panel 6/2(Pout) -> Add3/2
  PV Panel 5/1(Vout) -> Add1/1

== system PVRobusMPC_final/4 x 4 x 4 PV Panel 1/4 x 4 PV Panel 2/4 PV Panel 3 ==
  lambda_IR : Inport
  Tambient : Inport  Port=2
  Wind Speed : Inport  Port=3
  Add1 : Sum  Inputs=++++
  Add3 : Sum  Inputs=++++
  PV Panel 5 : Subsystem
  PV Panel 6 : Subsystem
  PV Panel 7 : Subsystem
  PV Panel 8 : Subsystem
  Vout : Outport
  Pout : Outport  Port=2
  wires:
  PV Panel 5/1(Vout) -> Add1/1
  PV Panel 6/2(Pout) -> Add3/2
  PV Panel 7/1(Vout) -> Add1/3
  Wind Speed/1 -> PV Panel 5/3(Wind Speed), PV Panel 6/3(Wind Speed), PV Panel 8/3(Wind Speed), PV Panel 7/3(Wind Speed)
  Tambient/1 -> PV Panel 5/2(Tambient), PV Panel 6/2(Tambient), PV Panel 8/2(Tambient), PV Panel 7/2(Tambient)
  Add3/1 -> Pout/1
  PV Panel 7/2(Pout) -> Add3/3
  lambda_IR/1 -> PV Panel 6/1(Lambda_IR), PV Panel 8/1(Lambda_IR), PV Panel 7/1(Lambda_IR), PV Panel 5/1(Lambda_IR)
  PV Panel 6/1(Vout) -> Add1/2
  PV Panel 8/1(Vout) -> Add1/4
  Add1/1 -> Vout/1
  PV Panel 8/2(Pout) -> Add3/4
  PV Panel 5/2(Pout) -> Add3/1

== system PVRobusMPC_final/4 x 4 x 4 PV Panel 1/4 x 4 PV Panel 2/4 PV Panel 4 ==
  lambda_IR : Inport
  Tambient : Inport  Port=2
  Wind Speed : Inport  Port=3
  Add1 : Sum  Inputs=++++
  Add3 : Sum  Inputs=++++
  PV Panel 5 : Subsystem
  PV Panel 6 : Subsystem
  PV Panel 7 : Subsystem
  PV Panel 8 : Subsystem
  Vout : Outport
  Pout : Outport  Port=2
  wires:
  PV Panel 5/2(Pout) -> Add3/1
  PV Panel 8/2(Pout) -> Add3/4
  Add1/1 -> Vout/1
  PV Panel 8/1(Vout) -> Add1/4
  PV Panel 6/1(Vout) -> Add1/2
  lambda_IR/1 -> PV Panel 5/1(Lambda_IR), PV Panel 7/1(Lambda_IR), PV Panel 8/1(Lambda_IR), PV Panel 6/1(Lambda_IR)
  PV Panel 7/2(Pout) -> Add3/3
  Add3/1 -> Pout/1
  Tambient/1 -> PV Panel 7/2(Tambient), PV Panel 8/2(Tambient), PV Panel 6/2(Tambient), PV Panel 5/2(Tambient)
  Wind Speed/1 -> PV Panel 7/3(Wind Speed), PV Panel 8/3(Wind Speed), PV Panel 6/3(Wind Speed), PV Panel 5/3(Wind Speed)
  PV Panel 7/1(Vout) -> Add1/3
  PV Panel 6/2(Pout) -> Add3/2
  PV Panel 5/1(Vout) -> Add1/1

== system PVRobusMPC_final/4 x 4 x 4 PV Panel 1/4 x 4 PV Panel 3/4 PV Panel 1 ==
  lambda_IR : Inport
  Tambient1 : Inport  Port=2
  Wind Speed : Inport  Port=3
  Add : Sum  Inputs=++++
  Add2 : Sum  Inputs=++++
  PV Panel 1 : Subsystem
  PV Panel 2 : Subsystem
  PV Panel 3 : Subsystem
  PV Panel 4 : Subsystem
  Vout : Outport
  Pout : Outport  Port=2
  wires:
  Add2/1 -> Pout/1
  PV Panel 2/1(Vout) -> Add/2
  PV Panel 4/2(Pout) -> Add2/4
  PV Panel 2/2(Pout) -> Add2/2
  PV Panel 3/1(Vout) -> Add/3
  Wind Speed/1 -> PV Panel 3/3(Wind Speed), PV Panel 4/3(Wind Speed), PV Panel 2/3(Wind Speed), PV Panel 1/3(Wind Speed)
  PV Panel 4/1(Vout) -> Add/4
  PV Panel 1/1(Vout) -> Add/1
  Tambient1/1 -> PV Panel 4/2(Tambient), PV Panel 3/2(Tambient), PV Panel 2/2(Tambient), PV Panel 1/2(Tambient)
  PV Panel 1/2(Pout) -> Add2/1
  Add/1 -> Vout/1
  lambda_IR/1 -> PV Panel 3/1(Lambda_IR), PV Panel 4/1(Lambda_IR), PV Panel 2/1(Lambda_IR), PV Panel 1/1(Lambda_IR)
  PV Panel 3/2(Pout) -> Add2/3

== system PVRobusMPC_final/4 x 4 x 4 PV Panel 1/4 x 4 PV Panel 3/4 PV Panel 2 ==
  lambda_IR : Inport
  Tambient : Inport  Port=2
  Wind Speed : Inport  Port=3
  Add1 : Sum  Inputs=++++
  Add3 : Sum  Inputs=++++
  PV Panel 5 : Subsystem
  PV Panel 6 : Subsystem
  PV Panel 7 : Subsystem
  PV Panel 8 : Subsystem
  Vout : Outport
  Pout : Outport  Port=2
  wires:
  PV Panel 5/2(Pout) -> Add3/1
  PV Panel 8/2(Pout) -> Add3/4
  Add1/1 -> Vout/1
  PV Panel 8/1(Vout) -> Add1/4
  PV Panel 6/1(Vout) -> Add1/2
  lambda_IR/1 -> PV Panel 5/1(Lambda_IR), PV Panel 7/1(Lambda_IR), PV Panel 8/1(Lambda_IR), PV Panel 6/1(Lambda_IR)
  PV Panel 7/2(Pout) -> Add3/3
  Add3/1 -> Pout/1
  Tambient/1 -> PV Panel 7/2(Tambient), PV Panel 8/2(Tambient), PV Panel 6/2(Tambient), PV Panel 5/2(Tambient)
  Wind Speed/1 -> PV Panel 7/3(Wind Speed), PV Panel 8/3(Wind Speed), PV Panel 6/3(Wind Speed), PV Panel 5/3(Wind Speed)
  PV Panel 7/1(Vout) -> Add1/3
  PV Panel 6/2(Pout) -> Add3/2
  PV Panel 5/1(Vout) -> Add1/1

== system PVRobusMPC_final/4 x 4 x 4 PV Panel 1/4 x 4 PV Panel 3/4 PV Panel 3 ==
  lambda_IR : Inport
  Tambient : Inport  Port=2
  Wind Speed : Inport  Port=3
  Add1 : Sum  Inputs=++++
  Add3 : Sum  Inputs=++++
  PV Panel 5 : Subsystem
  PV Panel 6 : Subsystem
  PV Panel 7 : Subsystem
  PV Panel 8 : Subsystem
  Vout : Outport
  Pout : Outport  Port=2
  wires:
  PV Panel 5/1(Vout) -> Add1/1
  PV Panel 6/2(Pout) -> Add3/2
  PV Panel 7/1(Vout) -> Add1/3
  Wind Speed/1 -> PV Panel 5/3(Wind Speed), PV Panel 6/3(Wind Speed), PV Panel 8/3(Wind Speed), PV Panel 7/3(Wind Speed)
  Tambient/1 -> PV Panel 5/2(Tambient), PV Panel 6/2(Tambient), PV Panel 8/2(Tambient), PV Panel 7/2(Tambient)
  Add3/1 -> Pout/1
  PV Panel 7/2(Pout) -> Add3/3
  lambda_IR/1 -> PV Panel 6/1(Lambda_IR), PV Panel 8/1(Lambda_IR), PV Panel 7/1(Lambda_IR), PV Panel 5/1(Lambda_IR)
  PV Panel 6/1(Vout) -> Add1/2
  PV Panel 8/1(Vout) -> Add1/4
  Add1/1 -> Vout/1
  PV Panel 8/2(Pout) -> Add3/4
  PV Panel 5/2(Pout) -> Add3/1

== system PVRobusMPC_final/4 x 4 x 4 PV Panel 1/4 x 4 PV Panel 3/4 PV Panel 4 ==
  lambda_IR : Inport
  Tambient : Inport  Port=2
  Wind Speed : Inport  Port=3
  Add1 : Sum  Inputs=++++
  Add3 : Sum  Inputs=++++
  PV Panel 5 : Subsystem
  PV Panel 6 : Subsystem
  PV Panel 7 : Subsystem
  PV Panel 8 : Subsystem
  Vout : Outport
  Pout : Outport  Port=2
  wires:
  PV Panel 5/2(Pout) -> Add3/1
  PV Panel 8/2(Pout) -> Add3/4
  Add1/1 -> Vout/1
  PV Panel 8/1(Vout) -> Add1/4
  PV Panel 6/1(Vout) -> Add1/2
  lambda_IR/1 -> PV Panel 5/1(Lambda_IR), PV Panel 7/1(Lambda_IR), PV Panel 8/1(Lambda_IR), PV Panel 6/1(Lambda_IR)
  PV Panel 7/2(Pout) -> Add3/3
  Add3/1 -> Pout/1
  Tambient/1 -> PV Panel 7/2(Tambient), PV Panel 8/2(Tambient), PV Panel 6/2(Tambient), PV Panel 5/2(Tambient)
  Wind Speed/1 -> PV Panel 7/3(Wind Speed), PV Panel 8/3(Wind Speed), PV Panel 6/3(Wind Speed), PV Panel 5/3(Wind Speed)
  PV Panel 7/1(Vout) -> Add1/3
  PV Panel 6/2(Pout) -> Add3/2
  PV Panel 5/1(Vout) -> Add1/1

== system PVRobusMPC_final/4 x 4 x 4 PV Panel 1/4 x 4 PV Panel 4/4 PV Panel 1 ==
  lambda_IR : Inport
  Tambient1 : Inport  Port=2
  Wind Speed : Inport  Port=3
  Add : Sum  Inputs=++++
  Add2 : Sum  Inputs=++++
  PV Panel 1 : Subsystem
  PV Panel 2 : Subsystem
  PV Panel 3 : Subsystem
  PV Panel 4 : Subsystem
  Vout : Outport
  Pout : Outport  Port=2
  wires:
  Add2/1 -> Pout/1
  PV Panel 2/1(Vout) -> Add/2
  PV Panel 4/2(Pout) -> Add2/4
  PV Panel 2/2(Pout) -> Add2/2
  PV Panel 3/1(Vout) -> Add/3
  Wind Speed/1 -> PV Panel 3/3(Wind Speed), PV Panel 4/3(Wind Speed), PV Panel 2/3(Wind Speed), PV Panel 1/3(Wind Speed)
  PV Panel 4/1(Vout) -> Add/4
  PV Panel 1/1(Vout) -> Add/1
  Tambient1/1 -> PV Panel 4/2(Tambient), PV Panel 3/2(Tambient), PV Panel 2/2(Tambient), PV Panel 1/2(Tambient)
  PV Panel 1/2(Pout) -> Add2/1
  Add/1 -> Vout/1
  lambda_IR/1 -> PV Panel 3/1(Lambda_IR), PV Panel 4/1(Lambda_IR), PV Panel 2/1(Lambda_IR), PV Panel 1/1(Lambda_IR)
  PV Panel 3/2(Pout) -> Add2/3

== system PVRobusMPC_final/4 x 4 x 4 PV Panel 1/4 x 4 PV Panel 4/4 PV Panel 2 ==
  lambda_IR : Inport
  Tambient : Inport  Port=2
  Wind Speed : Inport  Port=3
  Add1 : Sum  Inputs=++++
  Add3 : Sum  Inputs=++++
  PV Panel 5 : Subsystem
  PV Panel 6 : Subsystem
  PV Panel 7 : Subsystem
  PV Panel 8 : Subsystem
  Vout : Outport
  Pout : Outport  Port=2
  wires:
  PV Panel 5/2(Pout) -> Add3/1
  PV Panel 8/2(Pout) -> Add3/4
  Add1/1 -> Vout/1
  PV Panel 8/1(Vout) -> Add1/4
  PV Panel 6/1(Vout) -> Add1/2
  lambda_IR/1 -> PV Panel 5/1(Lambda_IR), PV Panel 7/1(Lambda_IR), PV Panel 8/1(Lambda_IR), PV Panel 6/1(Lambda_IR)
  PV Panel 7/2(Pout) -> Add3/3
  Add3/1 -> Pout/1
  Tambient/1 -> PV Panel 7/2(Tambient), PV Panel 8/2(Tambient), PV Panel 6/2(Tambient), PV Panel 5/2(Tambient)
  Wind Speed/1 -> PV Panel 7/3(Wind Speed), PV Panel 8/3(Wind Speed), PV Panel 6/3(Wind Speed), PV Panel 5/3(Wind Speed)
  PV Panel 7/1(Vout) -> Add1/3
  PV Panel 6/2(Pout) -> Add3/2
  PV Panel 5/1(Vout) -> Add1/1

== system PVRobusMPC_final/4 x 4 x 4 PV Panel 1/4 x 4 PV Panel 4/4 PV Panel 3 ==
  lambda_IR : Inport
  Tambient : Inport  Port=2
  Wind Speed : Inport  Port=3
  Add1 : Sum  Inputs=++++
  Add3 : Sum  Inputs=++++
  PV Panel 5 : Subsystem
  PV Panel 6 : Subsystem
  PV Panel 7 : Subsystem
  PV Panel 8 : Subsystem
  Vout : Outport
  Pout : Outport  Port=2
  wires:
  PV Panel 5/1(Vout) -> Add1/1
  PV Panel 6/2(Pout) -> Add3/2
  PV Panel 7/1(Vout) -> Add1/3
  Wind Speed/1 -> PV Panel 5/3(Wind Speed), PV Panel 6/3(Wind Speed), PV Panel 8/3(Wind Speed), PV Panel 7/3(Wind Speed)
  Tambient/1 -> PV Panel 5/2(Tambient), PV Panel 6/2(Tambient), PV Panel 8/2(Tambient), PV Panel 7/2(Tambient)
  Add3/1 -> Pout/1
  PV Panel 7/2(Pout) -> Add3/3
  lambda_IR/1 -> PV Panel 6/1(Lambda_IR), PV Panel 8/1(Lambda_IR), PV Panel 7/1(Lambda_IR), PV Panel 5/1(Lambda_IR)
  PV Panel 6/1(Vout) -> Add1/2
  PV Panel 8/1(Vout) -> Add1/4
  Add1/1 -> Vout/1
  PV Panel 8/2(Pout) -> Add3/4
  PV Panel 5/2(Pout) -> Add3/1

== system PVRobusMPC_final/4 x 4 x 4 PV Panel 1/4 x 4 PV Panel 4/4 PV Panel 4 ==
  lambda_IR : Inport
  Tambient : Inport  Port=2
  Wind Speed : Inport  Port=3
  Add1 : Sum  Inputs=++++
  Add3 : Sum  Inputs=++++
  PV Panel 5 : Subsystem
  PV Panel 6 : Subsystem
  PV Panel 7 : Subsystem
  PV Panel 8 : Subsystem
  Vout : Outport
  Pout : Outport  Port=2
  wires:
  PV Panel 5/2(Pout) -> Add3/1
  PV Panel 8/2(Pout) -> Add3/4
  Add1/1 -> Vout/1
  PV Panel 8/1(Vout) -> Add1/4
  PV Panel 6/1(Vout) -> Add1/2
  lambda_IR/1 -> PV Panel 5/1(Lambda_IR), PV Panel 7/1(Lambda_IR), PV Panel 8/1(Lambda_IR), PV Panel 6/1(Lambda_IR)
  PV Panel 7/2(Pout) -> Add3/3
  Add3/1 -> Pout/1
  Tambient/1 -> PV Panel 7/2(Tambient), PV Panel 8/2(Tambient), PV Panel 6/2(Tambient), PV Panel 5/2(Tambient)
  Wind Speed/1 -> PV Panel 7/3(Wind Speed), PV Panel 8/3(Wind Speed), PV Panel 6/3(Wind Speed), PV Panel 5/3(Wind Speed)
  PV Panel 7/1(Vout) -> Add1/3
  PV Panel 6/2(Pout) -> Add3/2
  PV Panel 5/1(Vout) -> Add1/1

== system PVRobusMPC_final/4 x 4 x 4 PV Panel 2/4 x 4 PV Panel 5/4 PV Panel 1 ==
  lambda_IR : Inport
  Tambient1 : Inport  Port=2
  Wind Speed : Inport  Port=3
  Add : Sum  Inputs=++++
  Add2 : Sum  Inputs=++++
  PV Panel 1 : Subsystem
  PV Panel 2 : Subsystem
  PV Panel 3 : Subsystem
  PV Panel 4 : Subsystem
  Vout : Outport
  Pout : Outport  Port=2
  wires:
  PV Panel 3/2(Pout) -> Add2/3
  lambda_IR/1 -> PV Panel 1/1(Lambda_IR), PV Panel 2/1(Lambda_IR), PV Panel 4/1(Lambda_IR), PV Panel 3/1(Lambda_IR)
  Add/1 -> Vout/1
  PV Panel 1/2(Pout) -> Add2/1
  Tambient1/1 -> PV Panel 1/2(Tambient), PV Panel 2/2(Tambient), PV Panel 3/2(Tambient), PV Panel 4/2(Tambient)
  PV Panel 1/1(Vout) -> Add/1
  PV Panel 4/1(Vout) -> Add/4
  Wind Speed/1 -> PV Panel 1/3(Wind Speed), PV Panel 2/3(Wind Speed), PV Panel 4/3(Wind Speed), PV Panel 3/3(Wind Speed)
  PV Panel 3/1(Vout) -> Add/3
  PV Panel 2/2(Pout) -> Add2/2
  PV Panel 4/2(Pout) -> Add2/4
  PV Panel 2/1(Vout) -> Add/2
  Add2/1 -> Pout/1

== system PVRobusMPC_final/4 x 4 x 4 PV Panel 2/4 x 4 PV Panel 5/4 PV Panel 2 ==
  lambda_IR : Inport
  Tambient : Inport  Port=2
  Wind Speed : Inport  Port=3
  Add1 : Sum  Inputs=++++
  Add3 : Sum  Inputs=++++
  PV Panel 5 : Subsystem
  PV Panel 6 : Subsystem
  PV Panel 7 : Subsystem
  PV Panel 8 : Subsystem
  Vout : Outport
  Pout : Outport  Port=2
  wires:
  PV Panel 5/1(Vout) -> Add1/1
  PV Panel 6/2(Pout) -> Add3/2
  PV Panel 7/1(Vout) -> Add1/3
  Wind Speed/1 -> PV Panel 5/3(Wind Speed), PV Panel 6/3(Wind Speed), PV Panel 8/3(Wind Speed), PV Panel 7/3(Wind Speed)
  Tambient/1 -> PV Panel 5/2(Tambient), PV Panel 6/2(Tambient), PV Panel 8/2(Tambient), PV Panel 7/2(Tambient)
  Add3/1 -> Pout/1
  PV Panel 7/2(Pout) -> Add3/3
  lambda_IR/1 -> PV Panel 6/1(Lambda_IR), PV Panel 8/1(Lambda_IR), PV Panel 7/1(Lambda_IR), PV Panel 5/1(Lambda_IR)
  PV Panel 6/1(Vout) -> Add1/2
  PV Panel 8/1(Vout) -> Add1/4
  Add1/1 -> Vout/1
  PV Panel 8/2(Pout) -> Add3/4
  PV Panel 5/2(Pout) -> Add3/1

== system PVRobusMPC_final/4 x 4 x 4 PV Panel 2/4 x 4 PV Panel 5/4 PV Panel 3 ==
  lambda_IR : Inport
  Tambient : Inport  Port=2
  Wind Speed : Inport  Port=3
  Add1 : Sum  Inputs=++++
  Add3 : Sum  Inputs=++++
  PV Panel 5 : Subsystem
  PV Panel 6 : Subsystem
  PV Panel 7 : Subsystem
  PV Panel 8 : Subsystem
  Vout : Outport
  Pout : Outport  Port=2
  wires:
  PV Panel 5/2(Pout) -> Add3/1
  PV Panel 8/2(Pout) -> Add3/4
  Add1/1 -> Vout/1
  PV Panel 8/1(Vout) -> Add1/4
  PV Panel 6/1(Vout) -> Add1/2
  lambda_IR/1 -> PV Panel 5/1(Lambda_IR), PV Panel 7/1(Lambda_IR), PV Panel 8/1(Lambda_IR), PV Panel 6/1(Lambda_IR)
  PV Panel 7/2(Pout) -> Add3/3
  Add3/1 -> Pout/1
  Tambient/1 -> PV Panel 7/2(Tambient), PV Panel 8/2(Tambient), PV Panel 6/2(Tambient), PV Panel 5/2(Tambient)
  Wind Speed/1 -> PV Panel 7/3(Wind Speed), PV Panel 8/3(Wind Speed), PV Panel 6/3(Wind Speed), PV Panel 5/3(Wind Speed)
  PV Panel 7/1(Vout) -> Add1/3
  PV Panel 6/2(Pout) -> Add3/2
  PV Panel 5/1(Vout) -> Add1/1

== system PVRobusMPC_final/4 x 4 x 4 PV Panel 2/4 x 4 PV Panel 5/4 PV Panel 4 ==
  lambda_IR : Inport
  Tambient : Inport  Port=2
  Wind Speed : Inport  Port=3
  Add1 : Sum  Inputs=++++
  Add3 : Sum  Inputs=++++
  PV Panel 5 : Subsystem
  PV Panel 6 : Subsystem
  PV Panel 7 : Subsystem
  PV Panel 8 : Subsystem
  Vout : Outport
  Pout : Outport  Port=2
  wires:
  PV Panel 5/1(Vout) -> Add1/1
  PV Panel 6/2(Pout) -> Add3/2
  PV Panel 7/1(Vout) -> Add1/3
  Wind Speed/1 -> PV Panel 5/3(Wind Speed), PV Panel 6/3(Wind Speed), PV Panel 8/3(Wind Speed), PV Panel 7/3(Wind Speed)
  Tambient/1 -> PV Panel 5/2(Tambient), PV Panel 6/2(Tambient), PV Panel 8/2(Tambient), PV Panel 7/2(Tambient)
  Add3/1 -> Pout/1
  PV Panel 7/2(Pout) -> Add3/3
  lambda_IR/1 -> PV Panel 6/1(Lambda_IR), PV Panel 8/1(Lambda_IR), PV Panel 7/1(Lambda_IR), PV Panel 5/1(Lambda_IR)
  PV Panel 6/1(Vout) -> Add1/2
  PV Panel 8/1(Vout) -> Add1/4
  Add1/1 -> Vout/1
  PV Panel 8/2(Pout) -> Add3/4
  PV Panel 5/2(Pout) -> Add3/1

== system PVRobusMPC_final/4 x 4 x 4 PV Panel 2/4 x 4 PV Panel 6/4 PV Panel 1 ==
  lambda_IR : Inport
  Tambient1 : Inport  Port=2
  Wind Speed : Inport  Port=3
  Add : Sum  Inputs=++++
  Add2 : Sum  Inputs=++++
  PV Panel 1 : Subsystem
  PV Panel 2 : Subsystem
  PV Panel 3 : Subsystem
  PV Panel 4 : Subsystem
  Vout : Outport
  Pout : Outport  Port=2
  wires:
  PV Panel 3/2(Pout) -> Add2/3
  lambda_IR/1 -> PV Panel 1/1(Lambda_IR), PV Panel 2/1(Lambda_IR), PV Panel 4/1(Lambda_IR), PV Panel 3/1(Lambda_IR)
  Add/1 -> Vout/1
  PV Panel 1/2(Pout) -> Add2/1
  Tambient1/1 -> PV Panel 1/2(Tambient), PV Panel 2/2(Tambient), PV Panel 3/2(Tambient), PV Panel 4/2(Tambient)
  PV Panel 1/1(Vout) -> Add/1
  PV Panel 4/1(Vout) -> Add/4
  Wind Speed/1 -> PV Panel 1/3(Wind Speed), PV Panel 2/3(Wind Speed), PV Panel 4/3(Wind Speed), PV Panel 3/3(Wind Speed)
  PV Panel 3/1(Vout) -> Add/3
  PV Panel 2/2(Pout) -> Add2/2
  PV Panel 4/2(Pout) -> Add2/4
  PV Panel 2/1(Vout) -> Add/2
  Add2/1 -> Pout/1

== system PVRobusMPC_final/4 x 4 x 4 PV Panel 2/4 x 4 PV Panel 6/4 PV Panel 2 ==
  lambda_IR : Inport
  Tambient : Inport  Port=2
  Wind Speed : Inport  Port=3
  Add1 : Sum  Inputs=++++
  Add3 : Sum  Inputs=++++
  PV Panel 5 : Subsystem
  PV Panel 6 : Subsystem
  PV Panel 7 : Subsystem
  PV Panel 8 : Subsystem
  Vout : Outport
  Pout : Outport  Port=2
  wires:
  PV Panel 5/1(Vout) -> Add1/1
  PV Panel 6/2(Pout) -> Add3/2
  PV Panel 7/1(Vout) -> Add1/3
  Wind Speed/1 -> PV Panel 5/3(Wind Speed), PV Panel 6/3(Wind Speed), PV Panel 8/3(Wind Speed), PV Panel 7/3(Wind Speed)
  Tambient/1 -> PV Panel 5/2(Tambient), PV Panel 6/2(Tambient), PV Panel 8/2(Tambient), PV Panel 7/2(Tambient)
  Add3/1 -> Pout/1
  PV Panel 7/2(Pout) -> Add3/3
  lambda_IR/1 -> PV Panel 6/1(Lambda_IR), PV Panel 8/1(Lambda_IR), PV Panel 7/1(Lambda_IR), PV Panel 5/1(Lambda_IR)
  PV Panel 6/1(Vout) -> Add1/2
  PV Panel 8/1(Vout) -> Add1/4
  Add1/1 -> Vout/1
  PV Panel 8/2(Pout) -> Add3/4
  PV Panel 5/2(Pout) -> Add3/1
